simulink model "modelo8_destilacion_perturbacion"  (R2014a)
settings: Solver=ode15s  StartTime=0.0  StopTime=10  RelTol=1e-3
values from neighbouring files (symbols this model uses):
  A = [-2.0500   -0.4000         0         0         0         0 ... (first row only)    [matrices_ejemplo.m]
  B = [1.0000         0 ... (first row only)    [matrices_ejemplo.m]
  C = [0.0719   -0.5752   -0.1594    0.6378         0         0 ... (first row only)    [matrices_ejemplo.m]
  Kff = inv(R)*B'*inv((A-B*K)')*Q*L    [matrices_ejemplo.m]
  Q2 = 40*eye(2)    [matrices_ejemplo.m]
  R = eye(2)    [matrices_ejemplo.m]
undefined symbols (not defined in the file or in its folder): K
settings Model: Creator=Juan Pablo Requez  LastModifiedBy=Juan Pablo Requez
settings DataIOCC: LimitDataPoints=off  SaveFormat=Dataset
settings OptimizationCC: SimCompilerOptimization=off
settings DebuggingCC: MergeDetectMultiDrivingBlocksExec=error  SolverPrmCheckMsg=none  FrameProcessingCompatibilityMsg=error
settings HardwareCC: ProdBitPerPointer=64  ProdLargestAtomicFloat=Float  ProdIntDivRoundTo=Zero  ProdEndianess=LittleEndian  ProdWordSize=64  ProdHWDeviceType=Intel->x86-64 (Windows64)
settings ModelReferenceCC: PropagateSignalLabelsOutOfModel=on
settings RTWCC: RTWCompilerOptimization=off
settings ConfigComp: CovMetricSettings=dw  CovHtmlReporting=on  CovSaveCumulativeToWorkspaceVar=on  CovSaveSingleToWorkspaceVar=on  CovExternalEMLEnable=off

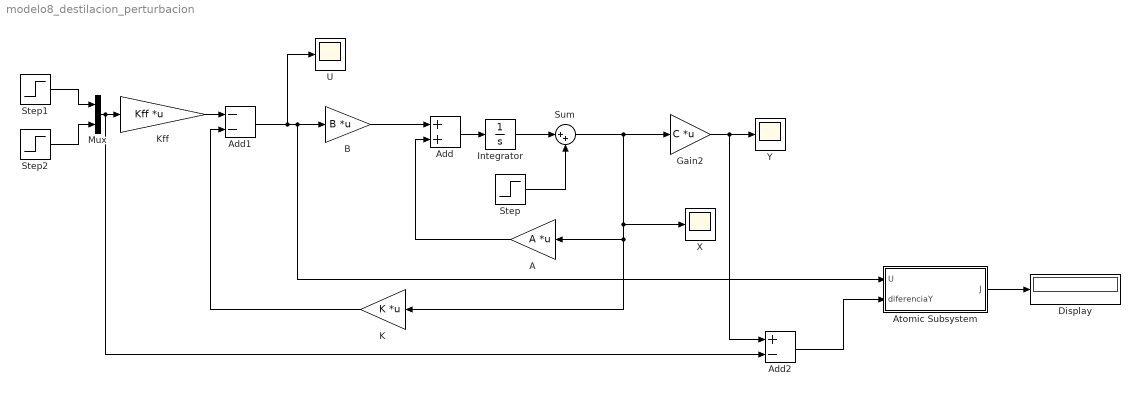
== system modelo8_destilacion_perturbacion ==
  A : Gain  Gain=A  Multiplication=Matrix(K*u)
  Add : Sum
  Add1 : Sum  Inputs=--
  Add2 : Sum  Inputs=+-
  Atomic Subsystem : Subsystem  TreatAsAtomicUnit=on
  B : Gain  Gain=B  Multiplication=Matrix(K*u)
  Display : Display
  Gain2 : Gain  Gain=C  Multiplication=Matrix(K*u)
  Integrator : Integrator
  K : Gain  Gain=K  Multiplication=Matrix(K*u)
  Kff : Gain  Gain=Kff  Multiplication=Matrix(K*u)
  Mux : Mux  Inputs=2
  Step : Step  Time=20  SampleTime=0
  Step1 : Step  Time=0  SampleTime=0
  Step2 : Step  Time=0  After=0  SampleTime=0
  Sum : Sum  Inputs=|++
  U : Scope
      settings: TimeRange=100  YMin=-2  YMax=0.5  SaveName=U
  X : Scope
      settings: SaveName=X
  Y : Scope
      settings: TimeRange=50  YMin=-0.1  YMax=0.7000000000000001  SaveName=Y
  wires:
  Add/1 -> Integrator/1
  B/1 -> Add/1
  A/1 -> Add/2
  Add1/1 -> U/1, Atomic Subsystem/1(U), B/1
  K/1 -> Add1/2
  Kff/1 -> Add1/1
  Gain2/1 -> Add2/1, Y/1
  Integrator/1 -> Sum/1
  Sum/1 -> X/1, K/1, A/1, Gain2/1
  Step/1 -> Sum/2
  Mux/1 -> Add2/2, Kff/1
  Step1/1 -> Mux/1
  Step2/1 -> Mux/2
  Atomic Subsystem/1(J) -> Display/1
  Add2/1 -> Atomic Subsystem/2(diferenciaY)

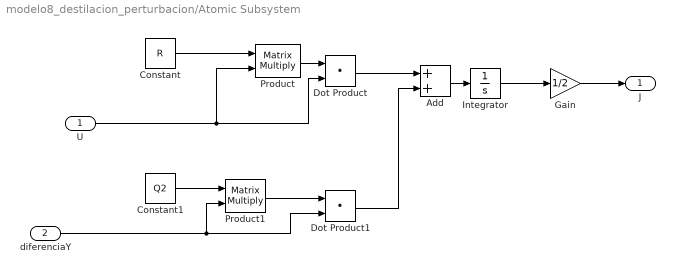
== system modelo8_destilacion_perturbacion/Atomic Subsystem ==
  U : Inport
  diferenciaY : Inport  Port=2
  Add : Sum
  Constant : Constant  Value=R
  Constant1 : Constant  Value=Q2
  Dot Product : DotProduct  InputSameDT=on  OutDataTypeStr=Inherit: Inherit via internal rule
  Dot Product1 : DotProduct  InputSameDT=on  OutDataTypeStr=Inherit: Inherit via internal rule
  Gain : Gain  Gain=1/2
  Integrator : Integrator
  Product : Product  Multiplication=Matrix(*)
  Product1 : Product  Multiplication=Matrix(*)
  J : Outport
  wires:
  U/1 -> Dot Product/2, Product/2
  Constant/1 -> Product/1
  Product/1 -> Dot Product/1
  Dot Product/1 -> Add/1
  Constant1/1 -> Product1/1
  diferenciaY/1 -> Dot Product1/2, Product1/2
  Product1/1 -> Dot Product1/1
  Dot Product1/1 -> Add/2
  Add/1 -> Integrator/1
  Integrator/1 -> Gain/1
  Gain/1 -> J/1
